simulink model "lookup_nD_TestGen24"  (R2017b)
settings: Solver=FixedStepDiscrete  StartTime=0.0  StopTime=10.0  RelTol=1e-3
model workspace (MAT data in the model file):
  LUTObjLKnD24 = Simulink.LookupTable
  LUTObjLKnD24.Table = Simulink.lookuptable.Table
  LUTObjLKnD24.Table.Value = reshape([4 16 10 4 16 10 5 19 18 5 19 18 6 20 23 6 20 23 7 21 24 7 21 24 8 22 25 8 22 25 4 16 10 4 16 10 5 19 18 5 19 18 6 20 23 6 20 23 7 21 24 7 21 24 8 22 25 8 22 25], [2 5 3 2])
  LUTObjLKnD24.Table.Dimensions = [2 5 3 2]
  LUTObjLKnD24.Table.DataType = 'auto'
  LUTObjLKnD24.Table.FieldName = 'Table'
  LUTObjLKnD24.BreakpointsSpecification = 'Even spacing'
  LUTObjLKnD24.Breakpoints(1) = Simulink.lookuptable.Evenspacing
  LUTObjLKnD24.Breakpoints(1).FirstPoint = 123.596514438
  LUTObjLKnD24.Breakpoints(1).Spacing = 1.5
  LUTObjLKnD24.Breakpoints(1).FirstPointName = 'BPFirstPoint1'
  LUTObjLKnD24.Breakpoints(1).SpacingName = 'BPSpacing1'
  LUTObjLKnD24.Breakpoints(1).TunableSizeName = 'N1'
  LUTObjLKnD24.Breakpoints(1).DataType = 'auto'
  LUTObjLKnD24.Breakpoints(1).FieldName = 'BP1'
  LUTObjLKnD24.Breakpoints(2) = Simulink.lookuptable.Evenspacing
  LUTObjLKnD24.Breakpoints(2).FirstPoint = 109.724037483
  LUTObjLKnD24.Breakpoints(2).Spacing = 1.5
  LUTObjLKnD24.Breakpoints(2).FirstPointName = 'BPFirstPoint2'
  LUTObjLKnD24.Breakpoints(2).SpacingName = 'BPSpacing2'
  LUTObjLKnD24.Breakpoints(2).TunableSizeName = 'N2'
  LUTObjLKnD24.Breakpoints(2).DataType = 'auto'
  LUTObjLKnD24.Breakpoints(2).FieldName = 'BP2'
  LUTObjLKnD24.Breakpoints(3) = Simulink.lookuptable.Evenspacing
  LUTObjLKnD24.Breakpoints(3).FirstPoint = 60.1097096414
  LUTObjLKnD24.Breakpoints(3).Spacing = 1.5
  LUTObjLKnD24.Breakpoints(3).FirstPointName = 'BPFirstPoint3'
  LUTObjLKnD24.Breakpoints(3).SpacingName = 'BPSpacing3'
  LUTObjLKnD24.Breakpoints(3).TunableSizeName = 'N3'
  LUTObjLKnD24.Breakpoints(3).DataType = 'auto'
  LUTObjLKnD24.Breakpoints(3).FieldName = 'BP3'
  LUTObjLKnD24.Breakpoints(4) = Simulink.lookuptable.Evenspacing
  LUTObjLKnD24.Breakpoints(4).FirstPoint = 115.152450412
  LUTObjLKnD24.Breakpoints(4).Spacing = 1.5
  LUTObjLKnD24.Breakpoints(4).FirstPointName = 'BPFirstPoint4'
  LUTObjLKnD24.Breakpoints(4).SpacingName = 'BPSpacing4'
  LUTObjLKnD24.Breakpoints(4).TunableSizeName = 'N4'
  LUTObjLKnD24.Breakpoints(4).DataType = 'auto'
  LUTObjLKnD24.Breakpoints(4).FieldName = 'BP4'
  LUTObjLKnD24.SupportTunableSize = 0
  LUTObjLKnD24.StructTypeInfo = Simulink.lookuptable.StructTypeInfo
  LUTObjLKnD24.StructTypeInfo.Name = 'LUT'
  LUTObjLKnD24.StructTypeInfo.DataScope = 'Auto'
undefined symbols (not defined in the file): Block_TestLib, enable
settings Model: Creator=ktrinh  LastModifiedBy=ktrinh
settings DebuggingCC: ParameterOverflowMsg=none

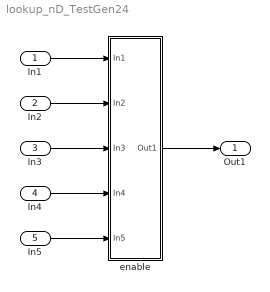
== system lookup_nD_TestGen24 ==
  In1 : Inport
  In2 : Inport  Port=2
  In3 : Inport  Port=3
  In4 : Inport  Port=4
  In5 : Inport  Port=5
  enable : Subsystem  AncestorBlock=Block_TestLib/enable
  Out1 : Outport
  wires:
  In1/1 -> enable/1(In1)
  In2/1 -> enable/2(In2)
  In3/1 -> enable/3(In3)
  In4/1 -> enable/4(In4)
  In5/1 -> enable/5(In5)
  enable/1(Out1) -> Out1/1

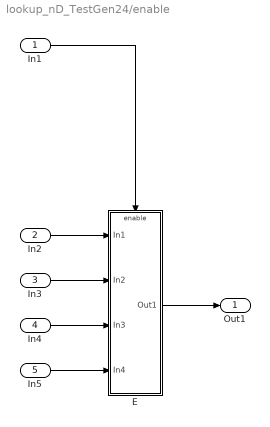
== system lookup_nD_TestGen24/enable ==
  In1 : Inport  OutDataTypeStr=boolean
  In2 : Inport  Port=2
  In3 : Inport  Port=3
  In4 : Inport  Port=4
  In5 : Inport  Port=5
  E : Subsystem  TreatAsAtomicUnit=on
  Out1 : Outport
  wires:
  In1/1 -> E/Enable
  In2/1 -> E/1(In1)
  In3/1 -> E/2(In2)
  In4/1 -> E/3(In3)
  In5/1 -> E/4(In4)
  E/1(Out1) -> Out1/1

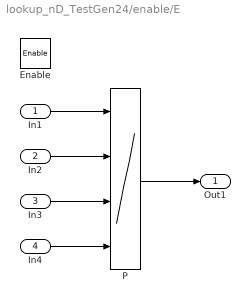
== system lookup_nD_TestGen24/enable/E ==
  In1 : Inport  OutMin=0  OutMax=127  PortDimensions=1
  In2 : Inport  Port=2  OutMin=0  OutMax=127
  In3 : Inport  Port=3  OutMin=0  OutMax=127
  In4 : Inport  Port=4  OutMin=0  OutMax=127
  Enable : EnablePort
  P : Lookup_n-D  NumberOfTableDimensions=4  DataSpecification=Lookup table object  LookupTableObject=LUTObjLKnD24  BreakpointsSpecification=Even spacing  BreakpointsForDimension3=[5, 7]  Table=reshape(repmat([4 5 6;16 19 20;10 18 23],1,2),[3,3,2])  UseLastTableValue=on  InternalRulePriority=Speed  RndMeth=Simplest  InputSameDT=on
  Out1 : Outport
  wires:
  In1/1 -> P/1
  In2/1 -> P/2
  In3/1 -> P/3
  In4/1 -> P/4
  P/1 -> Out1/1
